simulink model "NeuromuscularModelwReflex2"  (R2019b)
settings: Solver=ode15s  StartTime=0.0  StopTime=30  MaxStep=.01  RelTol=1e-4  AbsTol=1e-6  EnableMultiTasking=on
values from neighbouring files (symbols this model uses):
  LceOffsetTA = 1-0.5*w    [ControlParams.m]
  legAngleTgt = 1.2    [ControlParams.m]    (also in assignGains.m = Gains(45))
  LlegLengthClr = .9    (= 0.9)    [ControlParams.m]    (also in assignGains.m = Gains(20))
  LongDelay = 0.020    (= 0.02)    [ControlParams.m]
  MidDelay = 0.010    (= 0.01)    [ControlParams.m]
  RlegLengthClr = .9    (= 0.9)    [ControlParams.m]    (also in assignGains.m = Gains(41))
  ShortDelay = 0.005    [ControlParams.m]
  simbiconGainD = 5*pi/180    (= 0.0872664625997)    [ControlParams.m]    (also in assignGains.m = Gains(42))
  simbiconGainV = 5*pi/180    (= 0.0872664625997)    [ControlParams.m]    (also in assignGains.m = Gains(43))
  simbiconLegAngle0 = 85*pi/180    (= 1.4835298642)    [ControlParams.m]    (also in assignGains.m = Gains(44))
  termination_height = 0.5    [ControlParams.m]
undefined symbols (not defined in the file or in its folder): footCenterToCGDist, footInertia, footMass, g, loptGAS, loptHAM, loptHAMCut, loptTA, lslackGAS, lslackHAM, lslackHAMCut, phimaxGASa, phimaxGASk, phimaxHAMk, phirefGASa, phirefGASk, phirefHAMh, phirefHAMk, rGASa, rGASk, rHAMh, rHAMk, rhoGASa, rhoGASk, rhoHAMh, rhoHAMk, X, Y, Z
libraries: NeuroMuscularLibrary x86, nesl_utility x17, sm_lib x14, simulink x5, simulink_extras x2
(part 1 of 2)
settings Model: SimulationMode=rapid-accelerator  ParamWorkspaceSource=ReferencedWorkspace  ExtModeTrigDuration=100  TunableVars=LGainGAS,LGainGLU,LGainHAM,LGainKneeOverExt,LGainSOL,LGainSOLTA,LGainTA,LGainVAS,LKglu,LPosGainGG,LSpeedGainGG,LhipDGain,LhipPGain,LkneeExtendGain,LkneeFlexGain,LkneeHoldGain1,LkneeHoldGain2,LkneeStopGain,LlegAngleFilter,LlegLengthClr,PsimbiconGainD,PsimbiconGainV,PsimbiconLegAngle0,RGainGAS,RGainGLU,RGainHAM,RGainHAMCut,RGainKneeOverExt,RGainSOL,RGainSOLTA,RGainTA,RGainVAS,RKglu,RPosGainGG,RSpeedGainGG,RhipDGain,RhipPGain,RkneeExtendGain,RkneeFlexGain,RkneeHoldGain1,RkneeHoldGain2,RkneeStopGain,RlegAngleFilter,RlegLengthClr,ankleDgain,ankleFilterPID,ankleFilterSEA,anklePgain,groundTheta,groundX,groundZ,impulseTime,impulseValue,kneeDgain,kneeFilterPID,kneeFilterSEA,kneePgain,legAngleTgt,simbiconGainD,simbiconGainV,simbiconLegAngle0  TunableVarsStorageClass=Auto,Auto,Auto,Auto,Auto,Auto,Auto,Auto,Auto,Auto,Auto,Auto,Auto,Auto,Auto,Auto,Auto,Auto,Auto,Auto,Auto,Auto,Auto,Auto,Auto,Auto,Auto,Auto,Auto,Auto,Auto,Auto,Auto,Auto,Auto,Auto,Auto,Auto,Auto,Auto,Auto,Auto,Auto,Auto,Auto,Auto,Auto,Auto,Auto,Auto,Auto,Auto,Auto,Auto,Auto,Auto,Auto,Auto,Auto,Auto,Auto  TunableVarsTypeQualifier=,,,,,,,,,,,,,,,,,,,,,,,,,,,,,,,,,,,,,,,,,,,,,,,,,,,,,,,,,,,,  Creator=nitisht  LastModifiedBy=Nathan
settings SolverCC: AutoScaleAbsTol=off  ZeroCrossAlgorithm=Adaptive
settings DataIOCC: LimitDataPoints=on  SaveFinalState=on  SaveFormat=StructureWithTime  SaveOutput=off  SaveState=on  ReturnWorkspaceOutputs=off  StateSaveName=tmp_raccel_xout  SignalLoggingName=tmp_raccel_logsout
settings OptimizationCC: DefaultParameterBehavior=Inlined  InlineInvariantSignals=on  EnhancedBackFolding=on  EfficientMapNaN2IntZero=off  LifeSpan=inf  SimCompilerOptimization=on  AccelVerboseBuild=on
settings DebuggingCC: AlgebraicLoopMsg=error  SaveWithDisabledLinksMsg=none  UnderspecifiedInitializationDetection=Classic  MergeDetectMultiDrivingBlocksExec=none  TimeAdjustmentMsg=warning  MaskedZcDiagnostic=none  IgnoredZcDiagnostic=none  SolverPrmCheckMsg=warning  StateNameClashWarn=warning  SFUnexpectedBacktrackingDiag=warning  SFNoUnconditionalDefaultTransitionDiag=warning  SFExecutionAtInitializationDiag=none  ArithmeticOperatorsInVariantConditions=warning
settings HardwareCC: ProdBitPerLong=64  ProdLargestAtomicFloat=None  ProdHWDeviceType=Intel->x86-64  TargetBitPerPointer=64  TargetBitPerSizeT=64  TargetBitPerPtrDiffT=64  TargetLongLongMode=on  TargetIntDivRoundTo=Zero  TargetEndianess=LittleEndian  TargetWordSize=64  TargetHWDeviceType=MATLAB Host  ProdEqTarget=off
settings ModelReferenceCC: UpdateModelReferenceTargets=IfOutOfDate  PropagateSignalLabelsOutOfModel=off
settings SFSimCC: SFSimEcho=off  SimUseLocalCustomCode=off  CustomCodeUndefinedFunction=UseInterfaceOnly
settings RTWCC: SystemTargetFile=raccel.tlc  TemplateMakefile=raccel_default_tmf  RTWUseLocalCustomCode=off  RTWUseSimCustomCode=on
settings CodeAppCC: GenerateComments=off  MaxIdLength=128  MangleLength=10  SimulinkBlockComments=off
settings RaccelTargetCC: GeneratePreprocessorConditionals=Disable all  MultiInstanceERTCode=off  PreserveStateflowLocalDataDimensions=off  ENABLE_SLEXEC_SSBRIDGE=0  RTWCAPIParams=off
settings ConfigComp: CovMetricSettings=dw  CovHtmlReporting=on  CovSaveCumulativeToWorkspaceVar=on  CovSaveSingleToWorkspaceVar=on  CovExternalEMLEnable=off  CovSFcnEnable=off
settings SimscapeCC: SimscapeNormalizeSystem=off
settings ConfigurationSet: Description=SimMechanics 2G

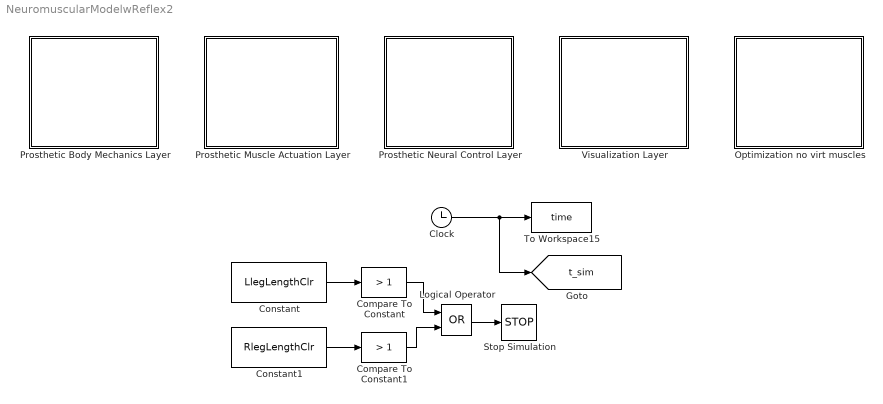
== system NeuromuscularModelwReflex2 ==
  Clock : Clock
  Compare To Constant : simulink/Logic and Bit Operations/Compare To Constant  relop=>  const=1  OutDataTypeStr=boolean
  Compare To Constant1 : simulink/Logic and Bit Operations/Compare To Constant  relop=>  const=1  OutDataTypeStr=boolean
  Constant : Constant  Value=LlegLengthClr
  Constant1 : Constant  Value=RlegLengthClr
  Logical Operator : Logic  Operator=OR  AllPortsSameDT=off  OutDataTypeStr=boolean
  Optimization no virt muscles : Subsystem
  Prosthetic Body Mechanics Layer : Subsystem
  Prosthetic Muscle Actuation Layer : Subsystem
  Prosthetic Neural Control Layer : Subsystem
  Stop Simulation : Stop
  To Workspace15 : ToWorkspace  VariableName=time  SampleTime=-1
      settings: MaxDataPoints=1
  Visualization Layer : Subsystem
  tag scope: t_sim=global
  wires:
  Clock/1 -> [t_sim], To Workspace15/1
  Compare To Constant/1 -> Logical Operator/1
  Logical Operator/1 -> Stop Simulation/1
  Compare To Constant1/1 -> Logical Operator/2
  Constant1/1 -> Compare To Constant1/1
  Constant/1 -> Compare To Constant/1

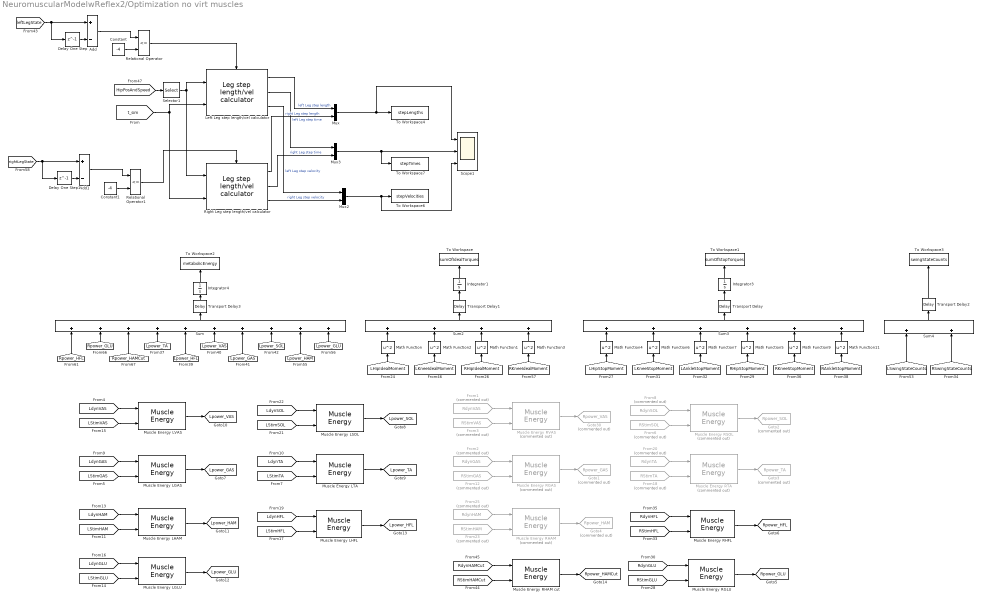
== system NeuromuscularModelwReflex2/Optimization no virt muscles ==
  Add : Sum  Inputs=+-
  Add1 : Sum  Inputs=+-
  Constant : Constant  Value=-4
  Constant1 : Constant  Value=-4
  Delay One Step : Delay  DelayLength=1
  Delay One Step1 : Delay  DelayLength=1
  From1 : From  Commented=on  GotoTag=RdynVAS  TagVisibility=global
  From12 : From  Commented=on  GotoTag=RStimGAS  TagVisibility=global
  From18 : From  Commented=on  GotoTag=RStimTA  TagVisibility=global
  From2 : From  Commented=on  GotoTag=RdynGAS  TagVisibility=global
  From20 : From  Commented=on  GotoTag=RdynTA  TagVisibility=global
  From23 : From  Commented=on  GotoTag=RStimHAM  TagVisibility=global
  From25 : From  Commented=on  GotoTag=RdynHAM  TagVisibility=global
  From3 : From  Commented=on  GotoTag=RStimVAS  TagVisibility=global
  From6 : From  Commented=on  GotoTag=RStimSOL  TagVisibility=global
  From8 : From  Commented=on  GotoTag=RdynSOL  TagVisibility=global
  Goto1 : Goto  Commented=on  GotoTag=Rpower_GAS  TagVisibility=global
  Goto2 : Goto  Commented=on  GotoTag=Rpower_SOL  TagVisibility=global
  Goto3 : Goto  Commented=on  GotoTag=Rpower_TA  TagVisibility=global
  Goto30 : Goto  Commented=on  GotoTag=Rpower_VAS  TagVisibility=global
  Goto4 : Goto  Commented=on  GotoTag=Rpower_HAM  TagVisibility=global
  Integrator1 : Integrator
  Integrator3 : Integrator
  Integrator4 : Integrator
  Left Leg step length/vel calculator : NeuroMuscularLibrary/Leg step length//vel calculator  SystemSampleTime=-1  Latency=0  AutoFrameSizeCalculation=off
  Math Function{,1..7,9,11} (10 alike) : Math  Operator=square  SaturateOnIntegerOverflow=on
  Muscle Energy LGAS : NeuroMuscularLibrary/Muscle Energy  lopt=loptGAS  FT=FT_GAS  Fmax=FmaxGAS
  Muscle Energy LGLU : NeuroMuscularLibrary/Muscle Energy  lopt=loptGLU  FT=FT_GLU  Fmax=FmaxGLU
  Muscle Energy LHAM : NeuroMuscularLibrary/Muscle Energy  lopt=loptHAM  FT=FT_HAM  Fmax=FmaxHAM
  Muscle Energy LHFL : NeuroMuscularLibrary/Muscle Energy  lopt=loptHFL  FT=FT_HFL  Fmax=FmaxHFL
  Muscle Energy LSOL : NeuroMuscularLibrary/Muscle Energy  lopt=loptSOL  FT=FT_SOL  Fmax=FmaxSOL
  Muscle Energy LTA : NeuroMuscularLibrary/Muscle Energy  lopt=loptTA  FT=FT_TA  Fmax=FmaxTA
  Muscle Energy LVAS : NeuroMuscularLibrary/Muscle Energy  lopt=loptVAS  FT=FT_VAS  Fmax=FmaxVAS
  Muscle Energy RGAS : NeuroMuscularLibrary/Muscle Energy  Commented=on  lopt=loptGAS  FT=FT_GAS  Fmax=FmaxGAS
  Muscle Energy RGLU : NeuroMuscularLibrary/Muscle Energy  lopt=loptGLU  FT=FT_GLU  Fmax=FmaxGLU
  Muscle Energy RHAM : NeuroMuscularLibrary/Muscle Energy  Commented=on  lopt=loptHAM  FT=FT_HAM  Fmax=FmaxHAM
  Muscle Energy RHAM cut : NeuroMuscularLibrary/Muscle Energy  lopt=loptHAMCut  FT=FT_HAM  Fmax=FmaxHAMCut
  Muscle Energy RHFL : NeuroMuscularLibrary/Muscle Energy  lopt=loptHFL  FT=FT_HFL  Fmax=FmaxHFL
  Muscle Energy RSOL : NeuroMuscularLibrary/Muscle Energy  Commented=on  lopt=loptSOL  FT=FT_SOL  Fmax=FmaxSOL
  Muscle Energy RTA : NeuroMuscularLibrary/Muscle Energy  Commented=on  lopt=loptTA  FT=FT_TA  Fmax=FmaxTA
  Muscle Energy RVAS : NeuroMuscularLibrary/Muscle Energy  Commented=on  lopt=loptVAS  FT=FT_VAS  Fmax=FmaxVAS
  Mux : Mux  Inputs=2
  Mux2 : Mux  Inputs=2
  Mux3 : Mux  Inputs=2
  Relational Operator : RelationalOperator  Operator=<=  OutDataTypeStr=boolean  RndMeth=Simplest
  Relational Operator1 : RelationalOperator  Operator=<=  OutDataTypeStr=boolean  RndMeth=Simplest
  Right Leg step length/vel calculator : NeuroMuscularLibrary/Leg step length//vel calculator  SystemSampleTime=-1  Latency=0  AutoFrameSizeCalculation=off
  Scope1 : Scope  NumInputPorts=3
  Selector1 : Selector  InputPortWidth=3  IndexOptions=Index vector (dialog)  Indices=[1]  OutputSizes=1
  Sum : Sum  Inputs=++++++++++
  Sum2 : Sum  Inputs=++++
  Sum3 : Sum  Inputs=++++++
  Sum4 : Sum
  To Workspace : ToWorkspace  VariableName=sumOfIdealTorques  SampleTime=-1
      settings: MaxDataPoints=1
  To Workspace1 : ToWorkspace  VariableName=sumOfStopTorques  SampleTime=-1
      settings: MaxDataPoints=1
  To Workspace2 : ToWorkspace  VariableName=metabolicEnergy  SampleTime=-1
      settings: MaxDataPoints=1
  To Workspace3 : ToWorkspace  VariableName=swingStateCounts  SampleTime=-1
      settings: MaxDataPoints=1
  To Workspace4 : ToWorkspace  VariableName=stepLengths  SampleTime=-1
  To Workspace6 : ToWorkspace  VariableName=stepVelocities  SampleTime=-1
  To Workspace7 : ToWorkspace  VariableName=stepTimes  SaveFormat=Structure With Time  SampleTime=-1
  Transport Delay{,1..3} (4 alike) : TransportDelay  DelayTime=3  BufferSize=24576
  tag scope: Lpower_GAS=global, Lpower_GLU=global, Lpower_HAM=global, Lpower_HFL=global, Lpower_SOL=global, Lpower_TA=global, Lpower_VAS=global, Rpower_GLU=global, Rpower_HAMCut=global, Rpower_HFL=global
  wires:
  Math Function5/1 -> Sum3/4
  Transport Delay1/1 -> Integrator1/1
  Sum2/1 -> Transport Delay1/1
  Transport Delay3/1 -> Integrator4/1
  Sum/1 -> Transport Delay3/1
  Integrator4/1 -> To Workspace2/1
  [Lpower_GAS] -> Sum/7
  [Lpower_SOL] -> Sum/8
  [Lpower_HAM] -> Sum/9
  [Lpower_GLU] -> Sum/10
  [Rpower_HAMCut] -> Sum/3
  [Lpower_TA] -> Sum/4
  [Lpower_HFL] -> Sum/5
  [Lpower_VAS] -> Sum/6
  [Rpower_GLU] -> Sum/2
  [Rpower_HFL] -> Sum/1
  [RSwingStateCounts] -> Sum4/2
  [LSwingStateCounts] -> Sum4/1
  Transport Delay2/1 -> To Workspace3/1
  Sum4/1 -> Transport Delay2/1
  Math Function11/1 -> Sum3/6
  [RAnkleStopMoment] -> Math Function11/1
  Math Function9/1 -> Sum3/5
  [RKneeStopMoment] -> Math Function9/1
  Transport Delay/1 -> Integrator3/1
  Sum3/1 -> Transport Delay/1
  [LAnkleStopMoment] -> Math Function7/1
  Math Function7/1 -> Sum3/3
  [RHipStopMoment] -> Math Function5/1
  [LKneeStopMoment] -> Math Function6/1
  Math Function6/1 -> Sum3/2
  [LHipStopMoment] -> Math Function4/1
  Math Function4/1 -> Sum3/1
  Integrator3/1 -> To Workspace1/1
  Math Function3/1 -> Sum2/4
  [RKneeIdealMoment] -> Math Function3/1
  Math Function1/1 -> Sum2/3
  [RHipIdealMoment] -> Math Function1/1
  [LKneeIdealMoment] -> Math Function2/1
  Math Function2/1 -> Sum2/2
  [LHipIdealMoment] -> Math Function/1
  Math Function/1 -> Sum2/1
  Integrator1/1 -> To Workspace/1
  Muscle Energy RHAM cut/1 -> [Rpower_HAMCut]
  [RStimHAMCut] -> Muscle Energy RHAM cut/2
  [RdynHAMCut] -> Muscle Energy RHAM cut/1
  [LdynVAS] -> Muscle Energy LVAS/1
  [LdynGAS] -> Muscle Energy LGAS/1
  Muscle Energy LHFL/1 -> [Lpower_HFL]
  Muscle Energy LGLU/1 -> [Lpower_GLU]
  Muscle Energy LHAM/1 -> [Lpower_HAM]
  [LStimHFL] -> Muscle Energy LHFL/2
  [LdynHFL] -> Muscle Energy LHFL/1
  [LStimGLU] -> Muscle Energy LGLU/2
  [LdynGLU] -> Muscle Energy LGLU/1
  [LStimHAM] -> Muscle Energy LHAM/2
  [LdynHAM] -> Muscle Energy LHAM/1
  [LStimTA] -> Muscle Energy LTA/2
  [LdynTA] -> Muscle Energy LTA/1
  Muscle Energy LTA/1 -> [Lpower_TA]
  Muscle Energy LSOL/1 -> [Lpower_SOL]
  Muscle Energy LGAS/1 -> [Lpower_GAS]
  Muscle Energy LVAS/1 -> [Lpower_VAS]
  [LStimGAS] -> Muscle Energy LGAS/2
  [LStimVAS] -> Muscle Energy LVAS/2
  [LStimSOL] -> Muscle Energy LSOL/2
  [LdynSOL] -> Muscle Energy LSOL/1
  From1/1 -> Muscle Energy RVAS/1
  From2/1 -> Muscle Energy RGAS/1
  Muscle Energy RHFL/1 -> [Rpower_HFL]
  Muscle Energy RGLU/1 -> [Rpower_GLU]
  Muscle Energy RHAM/1 -> Goto4/1
  [RStimHFL] -> Muscle Energy RHFL/2
  [RdynHFL] -> Muscle Energy RHFL/1
  [RStimGLU] -> Muscle Energy RGLU/2
  [RdynGLU] -> Muscle Energy RGLU/1
  From23/1 -> Muscle Energy RHAM/2
  From25/1 -> Muscle Energy RHAM/1
  From18/1 -> Muscle Energy RTA/2
  From20/1 -> Muscle Energy RTA/1
  Muscle Energy RTA/1 -> Goto3/1
  Muscle Energy RSOL/1 -> Goto2/1
  Muscle Energy RGAS/1 -> Goto1/1
  Muscle Energy RVAS/1 -> Goto30/1
  From12/1 -> Muscle Energy RGAS/2
  From3/1 -> Muscle Energy RVAS/2
  From6/1 -> Muscle Energy RSOL/2
  From8/1 -> Muscle Energy RSOL/1
  Mux3/1 -> Scope1/2, To Workspace7/1
  Right Leg step length/vel calculator/2 -> Mux3/2  "right Leg step time"
  Right Leg step length/vel calculator/3 -> Mux2/2  "right Leg step velocity"
  Left Leg step length/vel calculator/2 -> Mux3/1  "left Leg step time"
  [t_sim] -> Right Leg step length/vel calculator/2, Left Leg step length/vel calculator/2
  Left Leg step length/vel calculator/3 -> Mux2/1  "left Leg step velocity"
  Mux2/1 -> To Workspace6/1, Scope1/3
  Add1/1 -> Relational Operator1/1
  [leftLegState] -> Add/1, Delay One Step/1
  Delay One Step1/1 -> Add1/2
  Mux/1 -> To Workspace4/1, Scope1/1
  [rightLegState] -> Delay One Step1/1, Add1/1
  Relational Operator1/1 -> Right Leg step length/vel calculator/Enable
  Constant1/1 -> Relational Operator1/2
  Add/1 -> Relational Operator/1
  Delay One Step/1 -> Add/2
  Relational Operator/1 -> Left Leg step length/vel calculator/Enable
  Constant/1 -> Relational Operator/2
  Selector1/1 -> Right Leg step length/vel calculator/1, Left Leg step length/vel calculator/1
  Left Leg step length/vel calculator/1 -> Mux/1  "left Leg step length"
  [HipPosAndSpeed] -> Selector1/1
  Right Leg step length/vel calculator/1 -> Mux/2  "right Leg step length"

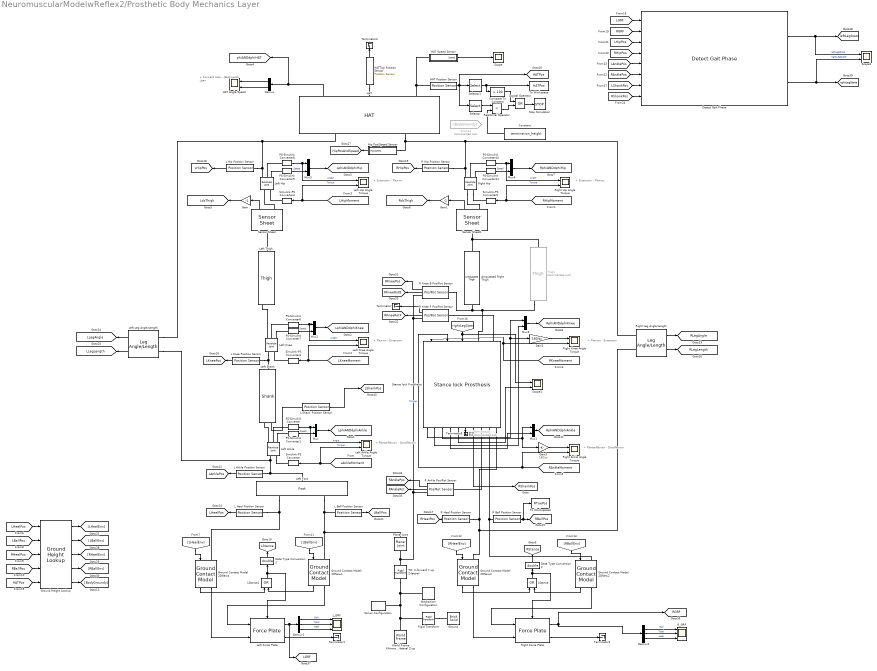
== system NeuromuscularModelwReflex2/Prosthetic Body Mechanics Layer ==
  note: + Plantarflexion
      | -  Dorsiflexion
  note: + Flexion
      | -  Extension
  note: + Extension
      | -  Flexion
  note: + Forward Lean
      | -  Backwards Lean
  note: + Extension
      | -  Flexion
  note: + Plantarflexion
      | -  Dorsiflexion
  note: + Flexion
      | -  Extension
  Amputated Right Thigh : NeuroMuscularLibrary/Amputated Thigh  SystemSampleTime=-1  Latency=0  AutoFrameSizeCalculation=off
  Compare To Constant : simulink/Logic and Bit Operations/Compare To Constant  relop=>  const=100  OutDataTypeStr=boolean
  Constant : Constant  Value=termination_height
  Data Type Conversion1 : DataTypeConversion  OutDataTypeStr=double
  Data Type Conversion2 : DataTypeConversion  OutDataTypeStr=double
  Demux : Demux  Outputs=2
  Demux1 : Demux  Outputs=3
  Demux2 : Demux  Outputs=3
  Detect Gait Phase : NeuroMuscularLibrary/Detect Gait Phase  SystemSampleTime=-1  Latency=0  AutoFrameSizeCalculation=off
  From14 : From  Commented=on  GotoTag=BodyGroundy
  Gain : Gain  Gain=-1
  Gain1 : Gain  Gain=-1
  Gain2 : Gain  Gain=180/pi
  Gain3 : Gain  Gain=180/pi
  Ground : sm_lib/Body Elements/Brick Solid  GraphicAmbientColor=[0.15 0.15 0.15 1.0]  BasedOnType=Density  BrickDimensions=[3 1 .01]  BrickDimensionUnits=m  CenterOfMass=[-footCenterToCGDist 0 0]  CenterOfMassUnits=m  GraphicDiffuseColor=[0.4 0.2 0.0]  Density=1000  DensityUnits=kg/(m^3)  DoExposeReferenceFrame=on  GraphicEmissiveColor=[0.0 0.0 0.0 1.0]  ExportEntireGeometry=off  SerializedFrames=<Frames/>  MarkerShape=Sphere  MarkerSize=10  GraphicType=FromGeometry  InertiaType=CalculateFromGeometry  Mass=footMass  MassUnits=kg  MomentsOfInertia=[0 0 footInertia]  MomentsOfInertiaUnits=kg*m^2  GraphicOpacity=1.0  ProductsOfInertia=[0 0 0]  ProductsOfInertiaUnits=kg*m^2  GraphicShininess=75  GraphicSpecularColor=[0.5 0.5 0.5 1.0]  GraphicVisPropType=SimpleVisualProperties
  Ground Contact Model 2DNew{1..4} (4 alike) : NeuroMuscularLibrary/Ground Contact Model  SystemSampleTime=-1  Latency=0  AutoFrameSizeCalculation=off
  Ground Height Lookup : NeuroMuscularLibrary/Ground Height Lookup  SystemSampleTime=-1  Latency=0  AutoFrameSizeCalculation=off
  HAT : NeuroMuscularLibrary/HAT  SystemSampleTime=-1  Latency=0  AutoFrameSizeCalculation=off
  HAT Position Sensor : NeuroMuscularLibrary/Position Sensor  SystemSampleTime=-1  Latency=0  AutoFrameSizeCalculation=off
  HAT Angle Speed : Scope  NumInputPorts=2
  HAT Speed Sensor : Subsystem
  HATTop Position Sensor : NeuroMuscularLibrary/Position Sensor  SystemSampleTime=-1  Latency=0  AutoFrameSizeCalculation=off
  Hip Pos/Speed Sensor : Subsystem
  L Ankle Position Sensor : NeuroMuscularLibrary/Position Sensor  SystemSampleTime=-1  Latency=0  AutoFrameSizeCalculation=off
  L Ball Position Sensor : NeuroMuscularLibrary/Position Sensor  SystemSampleTime=-1  Latency=0  AutoFrameSizeCalculation=off
  L Heel Position Sensor : NeuroMuscularLibrary/Position Sensor  SystemSampleTime=-1  Latency=0  AutoFrameSizeCalculation=off
  L Hip Position Sensor : NeuroMuscularLibrary/Position Sensor  SystemSampleTime=-1  Latency=0  AutoFrameSizeCalculation=off
  L Knee Position Sensor : NeuroMuscularLibrary/Position Sensor  SystemSampleTime=-1  Latency=0  AutoFrameSizeCalculation=off
  L Shank Position Sensor : NeuroMuscularLibrary/Position Sensor  SystemSampleTime=-1  Latency=0  AutoFrameSizeCalculation=off
  LStance : Logic  Operator=OR  AllPortsSameDT=off  OutDataTypeStr=boolean
  LStance1 : Logic  Operator=OR  AllPortsSameDT=off  OutDataTypeStr=boolean
  L_GRF : Scope  NumInputPorts=3
  Left Ankle : sm_lib/Joints/Revolute Joint  JointMode=Normal  SenseConstraintForce=off  SenseConstraintForceX=off  SenseConstraintForceY=off  SenseConstraintForceZ=off  SenseConstraintTorque=off  SenseConstraintTorqueX=off  SenseConstraintTorqueY=off  SenseConstraintTorqueZ=off  SenseTotalForce=off  SenseTotalForceX=off  SenseTotalForceY=off  SenseTotalForceZ=off  SenseTotalTorque=off  SenseTotalTorqueX=off  SenseTotalTorqueY=off  SenseTotalTorqueZ=off  CompositeWrenchDir=FollowerOnBase  CompositeWrenchFrame=BaseFrame  EquilibriumPosition=0  EquilibriumPositionUnits=deg  SpringStiffness=0  SpringStiffnessUnits=N*m/deg  DampingCoefficient=0  DampingCoefficientUnits=N*m/(deg/s)  TorqueActuationMode=InputTorque  MotionActuationMode=ComputedMotion  SensePosition=on  SenseVelocity=on  SenseAcceleration=off  SenseTorqueForce=off  SenseLowerLimitTorqueForce=off  SenseUpperLimitTorqueForce=off  LowerLimitSpecify=off  LowerLimitBound=-90  LowerLimitBoundUnits=deg  LowerLimitStiffness=1e4  LowerLimitStiffnessUnits=N*m/deg  LowerLimitDamping=10  LowerLimitDampingUnits=N*m/(deg/s)  LowerLimitTransitionRegionWidth=0.1  LowerLimitTransitionRegionWidthUnits=deg  UpperLimitSpecify=off  UpperLimitBound=90  UpperLimitBoundUnits=deg  UpperLimitStiffness=1e4  UpperLimitStiffnessUnits=N*m/deg  UpperLimitDamping=10  UpperLimitDampingUnits=N*m/(deg/s)  UpperLimitTransitionRegionWidth=0.1  UpperLimitTransitionRegionWidthUnits=deg  PositionTargetSpecify=on  PositionTargetPriority=High  PositionTargetValue=LphiAnkle0  PositionTargetValueUnits=rad  VelocityTargetSpecify=on  VelocityTargetPriority=Low  VelocityTargetValue=0  VelocityTargetValueUnits=rad/s
  Left Ankle Angle Torque : Scope  NumInputPorts=2
  Left Foot : NeuroMuscularLibrary/Foot  SystemSampleTime=-1  Latency=0  AutoFrameSizeCalculation=off
  Left Force Plate : NeuroMuscularLibrary/Force Plate  SystemSampleTime=-1  Latency=0  AutoFrameSizeCalculation=off
  Left Hip : sm_lib/Joints/Revolute Joint  JointMode=Normal  SenseConstraintForce=off  SenseConstraintForceX=off  SenseConstraintForceY=off  SenseConstraintForceZ=off  SenseConstraintTorque=off  SenseConstraintTorqueX=off  SenseConstraintTorqueY=off  SenseConstraintTorqueZ=off  SenseTotalForce=off  SenseTotalForceX=off  SenseTotalForceY=off  SenseTotalForceZ=off  SenseTotalTorque=off  SenseTotalTorqueX=off  SenseTotalTorqueY=off  SenseTotalTorqueZ=off  CompositeWrenchDir=FollowerOnBase  CompositeWrenchFrame=BaseFrame  EquilibriumPosition=0  EquilibriumPositionUnits=deg  SpringStiffness=0  SpringStiffnessUnits=N*m/deg  DampingCoefficient=0  DampingCoefficientUnits=N*m/(deg/s)  TorqueActuationMode=InputTorque  MotionActuationMode=ComputedMotion  SensePosition=on  SenseVelocity=on  SenseAcceleration=off  SenseTorqueForce=off  SenseLowerLimitTorqueForce=off  SenseUpperLimitTorqueForce=off  LowerLimitSpecify=off  LowerLimitBound=-90  LowerLimitBoundUnits=deg  LowerLimitStiffness=1e4  LowerLimitStiffnessUnits=N*m/deg  LowerLimitDamping=10  LowerLimitDampingUnits=N*m/(deg/s)  LowerLimitTransitionRegionWidth=0.1  LowerLimitTransitionRegionWidthUnits=deg  UpperLimitSpecify=off  UpperLimitBound=90  UpperLimitBoundUnits=deg  UpperLimitStiffness=1e4  UpperLimitStiffnessUnits=N*m/deg  UpperLimitDamping=10  UpperLimitDampingUnits=N*m/(deg/s)  UpperLimitTransitionRegionWidth=0.1  UpperLimitTransitionRegionWidthUnits=deg  PositionTargetSpecify=on  PositionTargetPriority=High  PositionTargetValue=LphiHip0  PositionTargetValueUnits=rad  VelocityTargetSpecify=on  VelocityTargetPriority=Low  VelocityTargetValue=0  VelocityTargetValueUnits=deg/s
  Left Hip Angle Torque : Scope  NumInputPorts=2
  Left Knee : sm_lib/Joints/Revolute Joint  JointMode=Normal  SenseConstraintForce=off  SenseConstraintForceX=off  SenseConstraintForceY=off  SenseConstraintForceZ=off  SenseConstraintTorque=off  SenseConstraintTorqueX=off  SenseConstraintTorqueY=off  SenseConstraintTorqueZ=off  SenseTotalForce=off  SenseTotalForceX=off  SenseTotalForceY=off  SenseTotalForceZ=off  SenseTotalTorque=off  SenseTotalTorqueX=off  SenseTotalTorqueY=off  SenseTotalTorqueZ=off  CompositeWrenchDir=FollowerOnBase  CompositeWrenchFrame=BaseFrame  EquilibriumPosition=0  EquilibriumPositionUnits=deg  SpringStiffness=0  SpringStiffnessUnits=N*m/deg  DampingCoefficient=0  DampingCoefficientUnits=N*m/(deg/s)  TorqueActuationMode=InputTorque  MotionActuationMode=ComputedMotion  SensePosition=on  SenseVelocity=on  SenseAcceleration=off  SenseTorqueForce=off  SenseLowerLimitTorqueForce=off  SenseUpperLimitTorqueForce=off  LowerLimitSpecify=off  LowerLimitBound=-90  LowerLimitBoundUnits=deg  LowerLimitStiffness=1e4  LowerLimitStiffnessUnits=N*m/deg  LowerLimitDamping=10  LowerLimitDampingUnits=N*m/(deg/s)  LowerLimitTransitionRegionWidth=0.1  LowerLimitTransitionRegionWidthUnits=deg  UpperLimitSpecify=off  UpperLimitBound=90  UpperLimitBoundUnits=deg  UpperLimitStiffness=1e4  UpperLimitStiffnessUnits=N*m/deg  UpperLimitDamping=10  UpperLimitDampingUnits=N*m/(deg/s)  UpperLimitTransitionRegionWidth=0.1  UpperLimitTransitionRegionWidthUnits=deg  PositionTargetSpecify=on  PositionTargetPriority=High  PositionTargetValue=LphiKnee0  PositionTargetValueUnits=rad  VelocityTargetSpecify=on  VelocityTargetPriority=Low  VelocityTargetValue=0  VelocityTargetValueUnits=deg/s
  Left Knee Angle Torque : Scope  NumInputPorts=2
  Left Leg Angle/Length : NeuroMuscularLibrary/Leg Angle//Length  SystemSampleTime=-1  Latency=0  AutoFrameSizeCalculation=off
  Left Shank : NeuroMuscularLibrary/Shank  SystemSampleTime=-1  Latency=0  AutoFrameSizeCalculation=off
  Left Thigh : NeuroMuscularLibrary/Thigh  SystemSampleTime=-1  Latency=0  AutoFrameSizeCalculation=off
  Logical Operator : Logic  Operator=OR  AllPortsSameDT=off  OutDataTypeStr=boolean
  Mechanism Configuration : sm_lib/Utilities/Mechanism Configuration  UniformGravity=Constant  GravityVector=[0 0 -g]  GravityUnits=m/s^2  LinearizationDelta=0.001
  Mux{,1..5} (6 alike) : Mux  Inputs=2
  PS-Simulink Converter{,6,8,10} (4 alike) : nesl_utility/PS-Simulink Converter  PhysicalDomain=network_engine_domain  SubClassName=ps_output  LeftPortType=input  RightPortType=output  PseudoPeriodic=off  Frequencies=[]  Unit=rad  AffineConversion=off
  PS-Simulink Converter{1,7,9,11} (4 alike) : nesl_utility/PS-Simulink Converter  PhysicalDomain=network_engine_domain  SubClassName=ps_output  LeftPortType=input  RightPortType=output  PseudoPeriodic=off  Frequencies=[]  Unit=rad/s  AffineConversion=off
  Planar Joint : sm_lib/Joints/Planar Joint  JointMode=Normal  SenseConstraintForce=off  SenseConstraintForceX=off  SenseConstraintForceY=off  SenseConstraintForceZ=off  SenseConstraintTorque=off  SenseConstraintTorqueX=off  SenseConstraintTorqueY=off  SenseConstraintTorqueZ=off  SenseTotalForce=off  SenseTotalForceX=off  SenseTotalForceY=off  SenseTotalForceZ=off  SenseTotalTorque=off  SenseTotalTorqueX=off  SenseTotalTorqueY=off  SenseTotalTorqueZ=off  CompositeWrenchDir=FollowerOnBase  CompositeWrenchFrame=BaseFrame  PxEquilibriumPosition=0  PxEquilibriumPositionUnits=m  PxSpringStiffness=0  PxSpringStiffnessUnits=N/m  PxDampingCoefficient=0  PxDampingCoefficientUnits=N/(m/s)  PxTorqueActuationMode=NoTorque  PxMotionActuationMode=ComputedMotion  PxSensePosition=off  PxSenseVelocity=off  PxSenseAcceleration=off  PxSenseTorqueForce=off  PxSenseLowerLimitTorqueForce=off  PxSenseUpperLimitTorqueForce=off  PxLowerLimitSpecify=off  PxLowerLimitBound=-1  PxLowerLimitBoundUnits=m  PxLowerLimitStiffness=1e6  PxLowerLimitStiffnessUnits=N/m  PxLowerLimitDamping=1e3  PxLowerLimitDampingUnits=N/(m/s)  PxLowerLimitTransitionRegionWidth=1e-4  PxLowerLimitTransitionRegionWidthUnits=m  PxUpperLimitSpecify=off  PxUpperLimitBound=1  PxUpperLimitBoundUnits=m  PxUpperLimitStiffness=1e6  PxUpperLimitStiffnessUnits=N/m  PxUpperLimitDamping=1e3  PxUpperLimitDampingUnits=N/(m/s)  PxUpperLimitTransitionRegionWidth=1e-4  PxUpperLimitTransitionRegionWidthUnits=m  PxPositionTargetSpecify=on  PxPositionTargetPriority=Low  PxPositionTargetValue=0  PxPositionTargetValueUnits=m  PxVelocityTargetSpecify=on  PxVelocityTargetPriority=High  PxVelocityTargetValue=vx0  PxVelocityTargetValueUnits=m/s  PyEquilibriumPosition=0  PyEquilibriumPositionUnits=m  PySpringStiffness=0  PySpringStiffnessUnits=N/m  PyDampingCoefficient=0  PyDampingCoefficientUnits=N/(m/s)  PyTorqueActuationMode=NoTorque  PyMotionActuationMode=ComputedMotion  PySensePosition=off  PySenseVelocity=off  PySenseAcceleration=off  PySenseTorqueForce=off  PySenseLowerLimitTorqueForce=off  PySenseUpperLimitTorqueForce=off  PyLowerLimitSpecify=off  PyLowerLimitBound=-1  PyLowerLimitBoundUnits=m  PyLowerLimitStiffness=1e6  PyLowerLimitStiffnessUnits=N/m  PyLowerLimitDamping=1e3  PyLowerLimitDampingUnits=N/(m/s)  PyLowerLimitTransitionRegionWidth=1e-4  PyLowerLimitTransitionRegionWidthUnits=m  PyUpperLimitSpecify=off  PyUpperLimitBound=1  PyUpperLimitBoundUnits=m  PyUpperLimitStiffness=1e6  PyUpperLimitStiffnessUnits=N/m  PyUpperLimitDamping=1e3  PyUpperLimitDampingUnits=N/(m/s)  PyUpperLimitTransitionRegionWidth=1e-4  PyUpperLimitTransitionRegionWidthUnits=m  PyPositionTargetSpecify=on  PyPositionTargetPriority=Low  PyPositionTargetValue=0  PyPositionTargetValueUnits=m  PyVelocityTargetSpecify=on  PyVelocityTargetPriority=Low  PyVelocityTargetValue=0  PyVelocityTargetValueUnits=m/s  RzEquilibriumPosition=0  RzEquilibriumPositionUnits=deg  RzSpringStiffness=0  RzSpringStiffnessUnits=N*m/deg  RzDampingCoefficient=0  RzDampingCoefficientUnits=N*m/(deg/s)  RzTorqueActuationMode=NoTorque  RzMotionActuationMode=ComputedMotion  RzSensePosition=off  RzSenseVelocity=off  RzSenseAcceleration=off  RzSenseTorqueForce=off  RzSenseLowerLimitTorqueForce=off  RzSenseUpperLimitTorqueForce=off  RzLowerLimitSpecify=off  RzLowerLimitBound=-90  RzLowerLimitBoundUnits=deg  RzLowerLimitStiffness=1e4  RzLowerLimitStiffnessUnits=N*m/deg  RzLowerLimitDamping=10  RzLowerLimitDampingUnits=N*m/(deg/s)  RzLowerLimitTransitionRegionWidth=0.1  RzLowerLimitTransitionRegionWidthUnits=deg  RzUpperLimitSpecify=off  RzUpperLimitBound=90  RzUpperLimitBoundUnits=deg  RzUpperLimitStiffness=1e4  RzUpperLimitStiffnessUnits=N*m/deg  RzUpperLimitDamping=10  RzUpperLimitDampingUnits=N*m/(deg/s)  RzUpperLimitTransitionRegionWidth=0.1  RzUpperLimitTransitionRegionWidthUnits=deg  RzPositionTargetSpecify=on  RzPositionTargetPriority=Low  RzPositionTargetValue=0  RzPositionTargetValueUnits=deg  RzVelocityTargetSpecify=on  RzVelocityTargetPriority=Low  RzVelocityTargetValue=0  RzVelocityTargetValueUnits=deg/s
  R Ankle Pos/Rot Sensor : NeuroMuscularLibrary/Pos//Rot Sensor  SystemSampleTime=-1  Latency=0  AutoFrameSizeCalculation=off
  R Ball Position Sensor : NeuroMuscularLibrary/Position Sensor  SystemSampleTime=-1  Latency=0  AutoFrameSizeCalculation=off
  R Heel Position Sensor : NeuroMuscularLibrary/Position Sensor  SystemSampleTime=-1  Latency=0  AutoFrameSizeCalculation=off
  R Hip Position Sensor : NeuroMuscularLibrary/Position Sensor  SystemSampleTime=-1  Latency=0  AutoFrameSizeCalculation=off
  R Knee B Pos/Rot Sensor : NeuroMuscularLibrary/Pos//Rot Sensor  SystemSampleTime=-1  Latency=0  AutoFrameSizeCalculation=off
  R Knee F Pos/Rot Sensor : NeuroMuscularLibrary/Pos//Rot Sensor  SystemSampleTime=-1  Latency=0  AutoFrameSizeCalculation=off
  R_GRF : Scope  NumInputPorts=3
  Relational Operator : RelationalOperator  Operator=<  OutDataTypeStr=boolean  RndMeth=Nearest
  Right Ankle Angle Torque : Scope  NumInputPorts=2
  Right Force Plate : NeuroMuscularLibrary/Force Plate  SystemSampleTime=-1  Latency=0  AutoFrameSizeCalculation=off
  Right Hip : sm_lib/Joints/Revolute Joint  JointMode=Normal  SenseConstraintForce=off  SenseConstraintForceX=off  SenseConstraintForceY=off  SenseConstraintForceZ=off  SenseConstraintTorque=off  SenseConstraintTorqueX=off  SenseConstraintTorqueY=off  SenseConstraintTorqueZ=off  SenseTotalForce=off  SenseTotalForceX=off  SenseTotalForceY=off  SenseTotalForceZ=off  SenseTotalTorque=off  SenseTotalTorqueX=off  SenseTotalTorqueY=off  SenseTotalTorqueZ=off  CompositeWrenchDir=FollowerOnBase  CompositeWrenchFrame=BaseFrame  EquilibriumPosition=0  EquilibriumPositionUnits=deg  SpringStiffness=0  SpringStiffnessUnits=N*m/deg  DampingCoefficient=0  DampingCoefficientUnits=N*m/(deg/s)  TorqueActuationMode=InputTorque  MotionActuationMode=ComputedMotion  SensePosition=on  SenseVelocity=on  SenseAcceleration=off  SenseTorqueForce=off  SenseLowerLimitTorqueForce=off  SenseUpperLimitTorqueForce=off  LowerLimitSpecify=off  LowerLimitBound=-90  LowerLimitBoundUnits=deg  LowerLimitStiffness=1e4  LowerLimitStiffnessUnits=N*m/deg  LowerLimitDamping=10  LowerLimitDampingUnits=N*m/(deg/s)  LowerLimitTransitionRegionWidth=0.1  LowerLimitTransitionRegionWidthUnits=deg  UpperLimitSpecify=off  UpperLimitBound=90  UpperLimitBoundUnits=deg  UpperLimitStiffness=1e4  UpperLimitStiffnessUnits=N*m/deg  UpperLimitDamping=10  UpperLimitDampingUnits=N*m/(deg/s)  UpperLimitTransitionRegionWidth=0.1  UpperLimitTransitionRegionWidthUnits=deg  PositionTargetSpecify=on  PositionTargetPriority=High  PositionTargetValue=RphiHip0  PositionTargetValueUnits=rad  VelocityTargetSpecify=on  VelocityTargetPriority=Low  VelocityTargetValue=0  VelocityTargetValueUnits=deg/s
  Right Hip Angle Torque : Scope  NumInputPorts=2
  Right Knee Angle Torque : Scope  NumInputPorts=2
  Right Leg Angle/Length : NeuroMuscularLibrary/Leg Angle//Length  SystemSampleTime=-1  Latency=0  AutoFrameSizeCalculation=off
  Rigid Transform : sm_lib/Frames and Transforms/Rigid Transform  TranslationMethod=Cartesian  TranslationStandardOffset=1  TranslationLengthUnit=m  TranslationStandardAxis=+X  TranslationCartesianOffset="[1  0 0]"  TranslationROffset=0  TranslationROffsetUnits=m  TranslationZOffset=0  TranslationZOffsetUnits=m  TranslationThetaOffset=0  TranslationThetaOffsetUnits=deg  RotationMethod=None  RotationAngleUnits=deg  RotationStandardAxis=+Z  RotationAngle=0  RotationArbitraryAxis=[0 0 1]  FollAlignAxisA=+X  BaseAlignAxisA=+Y  FollAlignAxisB=+Y  BaseAlignAxisB=+Z  RotationSequenceAxes=FollowerAxes  RotationSequence=XYX  RotationSequenceAngles=[0 0 0]  RotationSequenceAnglesUnits=deg  RotationMatrix=[1 0 0; 0 1 0; 0 0 1]
  Scope : Scope
  Scope1 : Scope  NumInputPorts=2
  Scope2 : Scope  NumInputPorts=2
  Selector : Selector  InputPortWidth=3  IndexOptions=Index vector (dialog)  Indices=[3]  OutputSizes=1
  Selector1 : Selector  InputPortWidth=3  IndexOptions=Index vector (dialog)  Indices=[1]  OutputSizes=1
  Sensor Sheet : NeuroMuscularLibrary/Sensor Sheet  SystemSampleTime=-1  Latency=0  AutoFrameSizeCalculation=off
  Sensor Sheet1 : NeuroMuscularLibrary/Sensor Sheet  SystemSampleTime=-1  Latency=0  AutoFrameSizeCalculation=off
  Simulink-PS Converter{,3..5} (4 alike) : nesl_utility/Simulink-PS Converter  PhysicalDomain=network_engine_domain  SubClassName=ps_input  LeftPortType=input  RightPortType=output  PseudoPeriodic=off  Frequencies=[]  NoiseDistribution=none  NoiseParameters=[]  Unit=N*m  AffineConversion=off  FilteringAndDerivatives=zero  SimscapeFilterOrder=1  InputFilterTimeConstant=0.001  UdotUserProvided=1
  Solver Configuration : nesl_utility/Solver Configuration  PhysicalDomain=network_engine_domain  SubClassName=solver  LeftPortType=input  RightPortType=generic  Tones=[]  Harmonics=[]  SimulateNoise=off  Profile=off  UseLocalSampling=off  EnableSwitchedLinearOptims=on  FrequencyDomain=off  UseCCode=off  RelTol=0.001  AbsTol=1e-06  MinStep=1e-09  ToWorkspace=off  RevertToSquareIcSolve=off  NumHomotopyIterations=100  PhasorMode=off  PhasorModeNumHarmonics=1  DoDC=off  ResidualTolerance=1e-09  UseLocalSolver=off  LocalSolverChoice=NE_BACKWARD_EULER_ADVANCER  LocalSolverSampleTime=0.001  DoFixedCost=off  MaxNonlinIter=3  MaxModeIter=2  LinearAlgebra=Sparse  EquationFormulation=NE_TIME_EF  DelaysMemoryBudget=1024  AutomaticFiltering=on  FilteringTimeConstant=0.001  PartitionStorageMethod=AS_NEEDED  PartitionMemoryBudget=1024  PartitionMethod=FAST
  Stance lock Prosthesis : NeuroMuscularLibrary/Stance lock Prosthesis  SystemSampleTime=-1  Latency=0  AutoFrameSizeCalculation=off
  Stop Simulation : Stop
  TO: X-forward Y-up Z-lateral : sm_lib/Frames and Transforms/Rigid Transform  TranslationMethod=StandardAxis  TranslationStandardOffset=hatLeftHipToCenterDistWidth  TranslationLengthUnit=m  TranslationStandardAxis=+Z  TranslationCartesianOffset=[0 0 0]  TranslationROffset=0  TranslationROffsetUnits=m  TranslationZOffset=0  TranslationZOffsetUnits=m  TranslationThetaOffset=0  TranslationThetaOffsetUnits=deg  RotationMethod=AlignedAxes  RotationAngleUnits=deg  RotationStandardAxis=+Z  RotationAngle=0  RotationArbitraryAxis=[0 0 1]  FollAlignAxisA=+Z  BaseAlignAxisA=+Y  FollAlignAxisB=+X  BaseAlignAxisB=+X  RotationSequenceAxes=FollowerAxes  RotationSequence=XYX  RotationSequenceAngles=[0 0 0]  RotationSequenceAnglesUnits=deg  RotationMatrix=[1 0 0; 0 1 0; 0 0 1]
  Terminator{,1..3,5} (5 alike) : Terminator
  Terminator4 : Terminator  Commented=on
  Thigh : NeuroMuscularLibrary/Thigh  Commented=on  SystemSampleTime=-1  Latency=0  AutoFrameSizeCalculation=off
  To Workspace : ToWorkspace  VariableName=HATPos  SampleTime=-1
      settings: MaxDataPoints=1
  To Workspace3 : ToWorkspace  VariableName=RToePos  SaveFormat=Structure With Time  SampleTime=-1
  World Frame X-forward Y-lateral Z-up : sm_lib/Frames and Transforms/World Frame
  tag scope: HATPos=global, HipPosAndSpeed=global, LAnklePos=global, LBallPos=global, LGRF=global, LHeelPos=global, LHipPos=global, LKneePos=global, LLegAngle=global, LLegLength=global, LShankPos=global, LStance=global, LdxThigh=global, LphiANDdphiAnkle=global, LphiANDdphiHip=global, LphiANDdphiKnee=global, RAnklePos=global, RAnkleRot=global, RBallPos=global, RGRF=global, RHeelPos=global, RHipPos=global, RKneePos=global, RKneeRotB=global, RKneeRotF=global, RLegAngle=global, RLegLength=global, RShankPos=global, RStance=global, RdxThigh=global, RphiANDdphiAnkle=global, RphiANDdphiHip=global, RphiANDdphiKnee=global, leftLegState=global, phiANDdphiHAT=global, rightLegState=global
  wires:
  Left Force Plate/1 -> [LGRF], Demux1/1
  Demux1/1 -> L_GRF/1  "Ball"
  Demux1/2 -> L_GRF/2  "Total"
  Demux1/3 -> L_GRF/3  "Heel"
  Left Force Plate/2 -> Terminator1/1
  Ground Contact Model 2DNew1/2 -> Left Force Plate/1
  Ground Contact Model 2DNew4/2 -> Left Force Plate/2
  Right Force Plate/1 -> [RGRF], Demux2/1
  Demux2/1 -> R_GRF/1  "Ball"
  Demux2/2 -> R_GRF/2  "Total"
  Demux2/3 -> R_GRF/3  "Heel"
  Right Force Plate/2 -> Terminator2/1
  Ground Contact Model 2DNew2/2 -> Right Force Plate/1
  Ground Contact Model 2DNew3/2 -> Right Force Plate/2
  LStance/1 -> Right Force Plate/Enable, Data Type Conversion2/1
  Mux/1 -> [LphiANDdphiAnkle]
  PS-Simulink Converter6/1 -> Left Knee Angle Torque/1, Mux2/1  "Angle"
  PS-Simulink Converter7/1 -> Mux2/2  "Speed"
  Demux/1 -> HAT Angle Speed/1
  PS-Simulink Converter/1 -> Left Ankle Angle Torque/1, Mux/1  "Angle"
  PS-Simulink Converter1/1 -> Mux/2  "Speed"
  Mux2/1 -> [LphiANDdphiKnee]
  [LKneeMoment] -> Simulink-PS Converter3/1, Left Knee Angle Torque/2
  Sensor Sheet/1 -> Gain/1
  PS-Simulink Converter9/1 -> Mux3/2  "Speed"
  HAT/1 -> [phiANDdphiHAT], Demux/1
  Demux/2 -> HAT Angle Speed/2
  Mux3/1 -> [LphiANDdphiHip]
  Gain/1 -> [LdxThigh]
  Sensor Sheet1/1 -> Gain1/1
  Gain1/1 -> [RdxThigh]
  Ground Contact Model 2DNew3/1 -> LStance/1
  Ground Contact Model 2DNew2/1 -> LStance/2
  LStance1/1 -> Left Force Plate/Enable, Data Type Conversion1/1
  Ground Contact Model 2DNew4/1 -> LStance1/1
  Ground Contact Model 2DNew1/1 -> LStance1/2
  Mux5/1 -> [RphiANDdphiKnee]
  Mux1/1 -> [RphiANDdphiAnkle]
  [RAnkleMoment] -> Stance lock Prosthesis/2, Right Ankle Angle Torque/2  "Torque"
  Mux4/1 -> [RphiANDdphiHip]
  L Ankle Position Sensor/1 -> [LAnklePos]
  L Heel Position Sensor/1 -> [LHeelPos]
  L Knee Position Sensor/1 -> [LKneePos]
  L Hip Position Sensor/1 -> [LHipPos]
  R Hip Position Sensor/1 -> [RHipPos]
  L Ball Position Sensor/1 -> [LBallPos]
  [RKneeMoment] -> Stance lock Prosthesis/1, Right Knee Angle Torque/2
  [LAnkleMoment] -> Simulink-PS Converter/1, Left Ankle Angle Torque/2  "Torque"
  [LHipMoment] -> Left Hip Angle Torque/2, Simulink-PS Converter4/1  "Torque"
  PS-Simulink Converter8/1 -> Left Hip Angle Torque/1, Mux3/1  "Angle"
  [RHipMoment] -> Right Hip Angle Torque/2, Simulink-PS Converter5/1  "Torque"
  PS-Simulink Converter10/1 -> Right Hip Angle Torque/1, Mux4/1  "Angle"
  PS-Simulink Converter11/1 -> Mux4/2  "Speed"
  Selector/1 -> Relational Operator/1
  Selector1/1 -> Compare To Constant/1, To Workspace/1
  Hip Pos/Speed Sensor/1(PosSpeed) -> [HipPosAndSpeed]
  Right Leg Angle/Length/1 -> [RLegAngle]
  Right Leg Angle/Length/2 -> [RLegLength]
  Left Leg Angle/Length/1 -> [LLegAngle]
  Left Leg Angle/Length/2 -> [LLegLength]
  Data Type Conversion1/1 -> [LStance]
  Data Type Conversion2/1 -> [RStance]
  R Ball Position Sensor/1 -> To Workspace3/1, [RBallPos]
  R Heel Position Sensor/1 -> [RHeelPos]
  [LHeelEnv] -> Ground Contact Model 2DNew4/1
  [LBallEnv] -> Ground Contact Model 2DNew1/1
  [RHeelEnv] -> Ground Contact Model 2DNew3/1
  [RBallEnv] -> Ground Contact Model 2DNew2/1
  R Knee F Pos/Rot Sensor/2 -> [RKneeRotF]
  R Knee B Pos/Rot Sensor/2 -> [RKneeRotB]
  R Knee B Pos/Rot Sensor/1 -> [RKneePos]
  R Ankle Pos/Rot Sensor/1 -> [RAnklePos]
  R Ankle Pos/Rot Sensor/2 -> [RAnkleRot]
  HAT Position Sensor/1 -> [HATPos], Selector/1, Selector1/1
  Compare To Constant/1 -> Logical Operator/1
  R Knee F Pos/Rot Sensor/1 -> Terminator/1
  Relational Operator/1 -> Logical Operator/2
  Logical Operator/1 -> Stop Simulation/1
  HATTop Position Sensor/1 -> Terminator3/1
  HAT Speed Sensor/1(Speed) -> Scope/1
  [LHeelPos] -> Ground Height Lookup/1
  Ground Height Lookup/1 -> [LHeelEnv]
  [LBallPos] -> Ground Height Lookup/2
  Ground Height Lookup/2 -> [LBallEnv]
  [RHeelPos] -> Ground Height Lookup/3
  Ground Height Lookup/3 -> [RHeelEnv]
  Ground Height Lookup/4 -> [RBallEnv]
  Ground Height Lookup/5 -> [BodyGroundy]
  [HATPos] -> Ground Height Lookup/5
  Stance lock Prosthesis/3 -> Gain3/1, Mux1/1
  Stance lock Prosthesis/4 -> Mux1/2
  Stance lock Prosthesis/2 -> Mux5/2
  Gain2/1 -> Right Knee Angle Torque/1
  Gain3/1 -> Right Ankle Angle Torque/1
  Stance lock Prosthesis/1 -> Gain2/1, Mux5/1
  Stance lock Prosthesis/5 -> Scope1/2
  Stance lock Prosthesis/6 -> Terminator5/1
  [RBallPos] -> Ground Height Lookup/4
  [rightLegState] -> Scope1/1, Stance lock Prosthesis/3
  [RHipPos] -> Detect Gait Phase/4
  [LAnklePos] -> Detect Gait Phase/5
  Detect Gait Phase/2 -> Scope2/2, [rightLegState]  "rightLegState"
  [RGRF] -> Detect Gait Phase/2
  [RShankPos] -> Detect Gait Phase/8
  [LHipPos] -> Detect Gait Phase/3
  [LShankPos] -> Detect Gait Phase/7
  [LGRF] -> Detect Gait Phase/1
  Detect Gait Phase/1 -> Scope2/1, [leftLegState]  "leftLegState"
  [RAnklePos] -> Detect Gait Phase/6
  Stance lock Prosthesis/7 -> [RShankPos]
  L Shank Position Sensor/1 -> [LShankPos]
  Constant/1 -> Relational Operator/2
  connections:
  TO: X-forward Y-up Z-lateral/RConn1 -- Mechanism Configuration/RConn1 -- Rigid Transform/LConn1 -- World Frame X-forward Y-lateral Z-up/RConn1 -- Solver Configuration/RConn1
  Left Ankle/RConn1 -- Left Shank/LConn1
  Left Ankle/RConn2 -- PS-Simulink Converter/LConn1
  Left Ankle/RConn3 -- PS-Simulink Converter1/LConn1
  Left Thigh/LConn1 -- Left Knee/RConn1
  Left Ankle/LConn2 -- Simulink-PS Converter/RConn1
  Simulink-PS Converter3/RConn1 -- Left Knee/LConn2
  Left Knee/RConn2 -- PS-Simulink Converter6/LConn1
  Left Knee/RConn3 -- PS-Simulink Converter7/LConn1
  Simulink-PS Converter4/RConn1 -- Left Hip/LConn2
  Left Hip/RConn2 -- PS-Simulink Converter8/LConn1
  Left Hip/RConn3 -- PS-Simulink Converter9/LConn1
  Rigid Transform/RConn1 -- Ground/RConn1
  Sensor Sheet/RConn1 -- Left Hip/LConn1
  Left Thigh/RConn1 -- Sensor Sheet/LConn1
  Amputated Right Thigh/RConn1 -- Thigh/RConn1 -- Sensor Sheet1/LConn1
  Right Hip/LConn1 -- Sensor Sheet1/RConn1
  Right Hip/LConn2 -- Simulink-PS Converter5/RConn1
  Right Hip/RConn3 -- PS-Simulink Converter11/LConn1
  Right Hip/RConn2 -- PS-Simulink Converter10/LConn1
  R Knee B Pos/Rot Sensor/LConn1 -- Thigh/LConn1 -- Stance lock Prosthesis/LConn1 -- Amputated Right Thigh/LConn1
  Ground Contact Model 2DNew2/LConn1 -- Stance lock Prosthesis/RConn2 -- R Ball Position Sensor/LConn1
  Left Hip/RConn1 -- L Hip Position Sensor/LConn1 -- Left Leg Angle/Length/LConn1 -- HAT/LConn1
  HAT/LConn2 -- Hip Pos/Speed Sensor/LConn1 -- Right Leg Angle/Length/LConn1 -- R Hip Position Sensor/LConn1 -- Right Hip/RConn1
  Left Knee/LConn1 -- L Knee Position Sensor/LConn1 -- Left Shank/RConn1
  Left Foot/LConn1 -- Ground Contact Model 2DNew4/LConn1 -- L Heel Position Sensor/LConn1
  Left Foot/LConn2 -- Ground Contact Model 2DNew1/LConn1 -- Planar Joint/RConn1 -- L Ball Position Sensor/LConn1
  R Knee F Pos/Rot Sensor/LConn1 -- Stance lock Prosthesis/LConn2
  HATTop Position Sensor/LConn1 -- HAT/RConn1
  Left Ankle/LConn1 -- Left Leg Angle/Length/LConn2 -- L Ankle Position Sensor/LConn1 -- Left Foot/RConn1
  R Knee B Pos/Rot Sensor/RConn1 -- R Ankle Pos/Rot Sensor/RConn1 -- Planar Joint/LConn1 -- TO: X-forward Y-up Z-lateral/LConn1 -- R Knee F Pos/Rot Sensor/RConn1
  HAT/RConn2 -- HAT Speed Sensor/LConn1 -- HAT Position Sensor/LConn1
  Right Leg Angle/Length/LConn2 -- Stance lock Prosthesis/RConn3 -- R Heel Position Sensor/LConn1 -- Ground Contact Model 2DNew3/LConn1
  Stance lock Prosthesis/RConn1 -- R Ankle Pos/Rot Sensor/LConn1
  L Shank Position Sensor/LConn1 -- Left Shank/LConn2
